simulink model "gimbal_test_2017_10_10"  (R2017a)
settings: Solver=ode14x  StartTime=0.0  StopTime=3  FixedStep=0.001  RelTol=1e-3  EnableMultiTasking=on
values from neighbouring files (symbols this model uses):
  m = MAG(:,3:5)    [acc_calibration_t1.m]
  s = tf('s')    [adaptive_control.m]    (also in constraints.m = 1e-19)
undefined symbols (not defined in the file or in its folder): sigbuilder_block, X, Y, Z
libraries: sm_lib x46, nesl_utility x29, simulink x7, sharedtransform x3
(part 2 of 2)

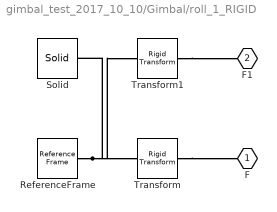
== system gimbal_test_2017_10_10/Gimbal/roll_1_RIGID ==
  ReferenceFrame : sm_lib/Frames and Transforms/Reference Frame
  Solid : sm_lib/Body Elements/Solid  InertiaType=Custom  Mass=0.31793228993235328  MassUnits=kg  CenterOfMass=[-40.197559372662035 151.39080125157062 -75.482343271011416]  CenterOfMassUnits=mm  MomentsOfInertia=[1698.578771208184 766.33943967936329 1161.8382457192142]  MomentsOfInertiaUnits=kg*mm^2  ProductsOfInertia=[-589.52899840909799 -20.442997774547614 -29.224073948839539]  ProductsOfInertiaUnits=kg*mm^2  DensityBased=on  Density=1000  DensityUnits=kg/(m^3)  DoExposeReferenceFrame=on  SerializedFrames=<Frames/>  GraphicType=FromGeometry  MarkerShape=Sphere  MarkerSize=10  GraphicVisPropType=SimpleVisualProperties  GraphicDiffuseColor=[0.89803921568627454 0.91764705882352937 0.92941176470588238]  GraphicSpecularColor=[0.5 0.5 0.5 1.0]  GraphicAmbientColor=[0.15 0.15 0.15 1.0]  GraphicEmissiveColor=[0.0 0.0 0.0 1.0]  GraphicShininess=75  GraphicOpacity=1  GeometryShape=FromFile  RectangleSize=[1 1]  RectangleSizeUnits=m  BrickDimensions=[1 1 1]  BrickDimensionUnits=m  CylinderRadius=1  CylinderRadiusUnits=m  CylinderLength=1  CylinderLengthUnits=m  SphereRadius=1  SphereRadiusUnits=m  EllipsoidRadii=[1 1 1]  EllipsoidRadiiUnits=m  ExtrusionCrossSection=[1 1; -1 1; -1 -1; 1 -1]  ExtrusionCrossSectionUnits=m  ExtrusionLength=1  ExtrusionLengthUnits=m  PolygonNumSides=3  PolygonOuterRadius=1  PolygonOuterRadiusUnits=m  ExtGeomFileType=STEP  ExtGeomFileName=roll_默认_sldprt.STEP  ExtGeomFileUnits=m  RevolutionCrossSection=[1 1; 1 -1; 2 -1; 2 1]  RevolutionCrossSectionUnits=m  RevolutionExtent=Full  RevolutionAngle=180  RevolutionAngleUnits=deg
  Transform : sm_lib/Frames and Transforms/Rigid Transform  TranslationMethod=Cartesian  TranslationStandardOffset=0  TranslationLengthUnit=mm  TranslationStandardAxis=+Z  TranslationCartesianOffset=[-38.909159672899136 47.175725301000313 513.35498149905948]  TranslationROffset=0  TranslationROffsetUnits=m  TranslationZOffset=0  TranslationZOffsetUnits=m  TranslationThetaOffset=0  TranslationThetaOffsetUnits=deg  RotationMethod=ArbitraryAxis  RotationAngleUnits=rad  RotationStandardAxis=+Z  RotationAngle=3.1415926535897931  RotationArbitraryAxis=[-1 1.5338031114433573e-32 -2.7175667253946204e-16]  FollAlignAxisA=+X  BaseAlignAxisA=+Y  FollAlignAxisB=+Y  BaseAlignAxisB=+Z  RotationSequenceAxes=FollowerAxes  RotationSequence=XYX  RotationSequenceAngles=[0 0 0]  RotationSequenceAnglesUnits=deg  RotationMatrix=[1 0 0; 0 1 0; 0 0 1]
  Transform1 : sm_lib/Frames and Transforms/Rigid Transform  TranslationMethod=Cartesian  TranslationStandardOffset=0  TranslationLengthUnit=mm  TranslationStandardAxis=+Z  TranslationCartesianOffset=[-38.909159672900039 1167.1810510685002 -32.030390597700006]  TranslationROffset=0  TranslationROffsetUnits=m  TranslationZOffset=0  TranslationZOffsetUnits=m  TranslationThetaOffset=0  TranslationThetaOffsetUnits=deg  RotationMethod=ArbitraryAxis  RotationAngleUnits=rad  RotationStandardAxis=+Z  RotationAngle=2.0943951023931953  RotationArbitraryAxis=[0.57735026918962584 -0.57735026918962584 0.57735026918962584]  FollAlignAxisA=+X  BaseAlignAxisA=+Y  FollAlignAxisB=+Y  BaseAlignAxisB=+Z  RotationSequenceAxes=FollowerAxes  RotationSequence=XYX  RotationSequenceAngles=[0 0 0]  RotationSequenceAnglesUnits=deg  RotationMatrix=[1 0 0; 0 1 0; 0 0 1]
  F : PMIOPort  Port=1  Side=Left
  F1 : PMIOPort  Port=2  Side=Right
  connections:
  Solid/RConn1 -- ReferenceFrame/RConn1 -- Transform/LConn1 -- Transform1/LConn1
  Transform/RConn1 -- F/RConn1
  Transform1/RConn1 -- F1/RConn1

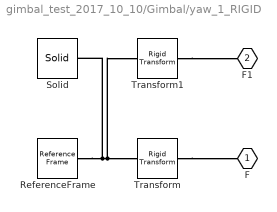
== system gimbal_test_2017_10_10/Gimbal/yaw_1_RIGID ==
  ReferenceFrame : sm_lib/Frames and Transforms/Reference Frame
  Solid : sm_lib/Body Elements/Solid  InertiaType=Custom  Mass=0.4220224652422469  MassUnits=kg  CenterOfMass=[-39.730395407906954 147.5203430562342 -125.35459490281445]  CenterOfMassUnits=mm  MomentsOfInertia=[6109.2729904538583 920.66918616811347 5510.6384164735264]  MomentsOfInertiaUnits=kg*mm^2  ProductsOfInertia=[-1282.9600428246124 21.67357327564007 52.078346871971853]  ProductsOfInertiaUnits=kg*mm^2  DensityBased=on  Density=1000  DensityUnits=kg/(m^3)  DoExposeReferenceFrame=on  SerializedFrames=<Frames/>  GraphicType=FromGeometry  MarkerShape=Sphere  MarkerSize=10  GraphicVisPropType=SimpleVisualProperties  GraphicDiffuseColor=[0.89803921568627454 0.91764705882352937 0.92941176470588238]  GraphicSpecularColor=[0.5 0.5 0.5 1.0]  GraphicAmbientColor=[0.15 0.15 0.15 1.0]  GraphicEmissiveColor=[0.0 0.0 0.0 1.0]  GraphicShininess=75  GraphicOpacity=1  GeometryShape=FromFile  RectangleSize=[1 1]  RectangleSizeUnits=m  BrickDimensions=[1 1 1]  BrickDimensionUnits=m  CylinderRadius=1  CylinderRadiusUnits=m  CylinderLength=1  CylinderLengthUnits=m  SphereRadius=1  SphereRadiusUnits=m  EllipsoidRadii=[1 1 1]  EllipsoidRadiiUnits=m  ExtrusionCrossSection=[1 1; -1 1; -1 -1; 1 -1]  ExtrusionCrossSectionUnits=m  ExtrusionLength=1  ExtrusionLengthUnits=m  PolygonNumSides=3  PolygonOuterRadius=1  PolygonOuterRadiusUnits=m  ExtGeomFileType=STEP  ExtGeomFileName=yaw_默认_sldprt.STEP  ExtGeomFileUnits=m  RevolutionCrossSection=[1 1; 1 -1; 2 -1; 2 1]  RevolutionCrossSectionUnits=m  RevolutionExtent=Full  RevolutionAngle=180  RevolutionAngleUnits=deg
  Transform : sm_lib/Frames and Transforms/Rigid Transform  TranslationMethod=Cartesian  TranslationStandardOffset=0  TranslationLengthUnit=mm  TranslationStandardAxis=+Z  TranslationCartesianOffset=[-38.909159672899804 334.03951901900109 -32.030390597700091]  TranslationROffset=0  TranslationROffsetUnits=m  TranslationZOffset=0  TranslationZOffsetUnits=m  TranslationThetaOffset=0  TranslationThetaOffsetUnits=deg  RotationMethod=ArbitraryAxis  RotationAngleUnits=rad  RotationStandardAxis=+Z  RotationAngle=2.0943951023931962  RotationArbitraryAxis=[0.57735026918962595 -0.57735026918962562 0.57735026918962573]  FollAlignAxisA=+X  BaseAlignAxisA=+Y  FollAlignAxisB=+Y  BaseAlignAxisB=+Z  RotationSequenceAxes=FollowerAxes  RotationSequence=XYX  RotationSequenceAngles=[0 0 0]  RotationSequenceAnglesUnits=deg  RotationMatrix=[1 0 0; 0 1 0; 0 0 1]
  Transform1 : sm_lib/Frames and Transforms/Rigid Transform  TranslationMethod=Cartesian  TranslationStandardOffset=0  TranslationLengthUnit=mm  TranslationStandardAxis=+Z  TranslationCartesianOffset=[-38.909159672900067 32.039519019000039 520.28895609530014]  TranslationROffset=0  TranslationROffsetUnits=m  TranslationZOffset=0  TranslationZOffsetUnits=m  TranslationThetaOffset=0  TranslationThetaOffsetUnits=deg  RotationMethod=ArbitraryAxis  RotationAngleUnits=rad  RotationStandardAxis=+Z  RotationAngle=3.1415926535897931  RotationArbitraryAxis=[1 0 5.377642775528102e-17]  FollAlignAxisA=+X  BaseAlignAxisA=+Y  FollAlignAxisB=+Y  BaseAlignAxisB=+Z  RotationSequenceAxes=FollowerAxes  RotationSequence=XYX  RotationSequenceAngles=[0 0 0]  RotationSequenceAnglesUnits=deg  RotationMatrix=[1 0 0; 0 1 0; 0 0 1]
  F : PMIOPort  Port=1  Side=Left
  F1 : PMIOPort  Port=2  Side=Right
  connections:
  Solid/RConn1 -- ReferenceFrame/RConn1 -- Transform/LConn1 -- Transform1/LConn1
  Transform/RConn1 -- F/RConn1
  Transform1/RConn1 -- F1/RConn1

== system gimbal_test_2017_10_10/Subsystem1/groud_1_RIGID ==
  ReferenceFrame : sm_lib/Frames and Transforms/Reference Frame
  Solid : sm_lib/Body Elements/Solid  InertiaType=Custom  Mass=0.744656095436107  MassUnits=kg  CenterOfMass=[0 14.834199182049298 0]  CenterOfMassUnits=mm  MomentsOfInertia=[248.52962199765179 383.88524366097863 245.75166872905808]  MomentsOfInertiaUnits=kg*mm^2  ProductsOfInertia=[0 0 0]  ProductsOfInertiaUnits=kg*mm^2  DensityBased=on  Density=1000  DensityUnits=kg/(m^3)  DoExposeReferenceFrame=on  SerializedFrames=<Frames/>  GraphicType=FromGeometry  MarkerShape=Sphere  MarkerSize=10  GraphicVisPropType=SimpleVisualProperties  GraphicDiffuseColor=[0.89411764705882346 0.9137254901960784 0.92941176470588238]  GraphicSpecularColor=[0.5 0.5 0.5 1.0]  GraphicAmbientColor=[0.15 0.15 0.15 1.0]  GraphicEmissiveColor=[0.0 0.0 0.0 1.0]  GraphicShininess=75  GraphicOpacity=1  GeometryShape=FromFile  RectangleSize=[1 1]  RectangleSizeUnits=m  BrickDimensions=[1 1 1]  BrickDimensionUnits=m  CylinderRadius=1  CylinderRadiusUnits=m  CylinderLength=1  CylinderLengthUnits=m  SphereRadius=1  SphereRadiusUnits=m  EllipsoidRadii=[1 1 1]  EllipsoidRadiiUnits=m  ExtrusionCrossSection=[1 1; -1 1; -1 -1; 1 -1]  ExtrusionCrossSectionUnits=m  ExtrusionLength=1  ExtrusionLengthUnits=m  PolygonNumSides=3  PolygonOuterRadius=1  PolygonOuterRadiusUnits=m  ExtGeomFileType=STEP  ExtGeomFileName=groud_默认_sldprt.STEP  ExtGeomFileUnits=m  RevolutionCrossSection=[1 1; 1 -1; 2 -1; 2 1]  RevolutionCrossSectionUnits=m  RevolutionExtent=Full  RevolutionAngle=180  RevolutionAngleUnits=deg
  Transform : sm_lib/Frames and Transforms/Rigid Transform  TranslationMethod=Cartesian  TranslationStandardOffset=0  TranslationLengthUnit=mm  TranslationStandardAxis=+Z  TranslationCartesianOffset=[0 30 0]  TranslationROffset=0  TranslationROffsetUnits=m  TranslationZOffset=0  TranslationZOffsetUnits=m  TranslationThetaOffset=0  TranslationThetaOffsetUnits=deg  RotationMethod=ArbitraryAxis  RotationAngleUnits=rad  RotationStandardAxis=+Z  RotationAngle=2.0943951023931953  RotationArbitraryAxis=[0.57735026918962584 -0.57735026918962584 0.57735026918962584]  FollAlignAxisA=+X  BaseAlignAxisA=+Y  FollAlignAxisB=+Y  BaseAlignAxisB=+Z  RotationSequenceAxes=FollowerAxes  RotationSequence=XYX  RotationSequenceAngles=[0 0 0]  RotationSequenceAnglesUnits=deg  RotationMatrix=[1 0 0; 0 1 0; 0 0 1]
  F1 : PMIOPort  Port=1  Side=Left
  F : PMIOPort  Port=2  Side=Right
  connections:
  Solid/RConn1 -- ReferenceFrame/RConn1 -- Transform/LConn1 -- F1/RConn1
  Transform/RConn1 -- F/RConn1

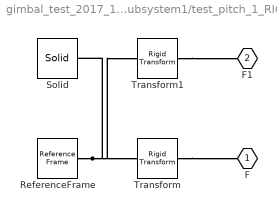
== system gimbal_test_2017_10_10/Subsystem1/test_pitch_1_RIGID ==
  ReferenceFrame : sm_lib/Frames and Transforms/Reference Frame
  Solid : sm_lib/Body Elements/Solid  InertiaType=Custom  Mass=3.2542558482698221  MassUnits=kg  CenterOfMass=[0 15.000000000000004 0.00013445046945364221]  CenterOfMassUnits=mm  MomentsOfInertia=[197323.97689125084 354318.98035563418 157585.85549691919]  MomentsOfInertiaUnits=kg*mm^2  ProductsOfInertia=[0 0 0.0039657370023979469]  ProductsOfInertiaUnits=kg*mm^2  DensityBased=on  Density=1000  DensityUnits=kg/(m^3)  DoExposeReferenceFrame=on  SerializedFrames=<Frames/>  GraphicType=FromGeometry  MarkerShape=Sphere  MarkerSize=10  GraphicVisPropType=SimpleVisualProperties  GraphicDiffuseColor=[1 1 1]  GraphicSpecularColor=[0.5 0.5 0.5 1.0]  GraphicAmbientColor=[0.15 0.15 0.15 1.0]  GraphicEmissiveColor=[0.0 0.0 0.0 1.0]  GraphicShininess=75  GraphicOpacity=1  GeometryShape=FromFile  RectangleSize=[1 1]  RectangleSizeUnits=m  BrickDimensions=[1 1 1]  BrickDimensionUnits=m  CylinderRadius=1  CylinderRadiusUnits=m  CylinderLength=1  CylinderLengthUnits=m  SphereRadius=1  SphereRadiusUnits=m  EllipsoidRadii=[1 1 1]  EllipsoidRadiiUnits=m  ExtrusionCrossSection=[1 1; -1 1; -1 -1; 1 -1]  ExtrusionCrossSectionUnits=m  ExtrusionLength=1  ExtrusionLengthUnits=m  PolygonNumSides=3  PolygonOuterRadius=1  PolygonOuterRadiusUnits=m  ExtGeomFileType=STEP  ExtGeomFileName=test_pitch_默认_sldprt.STEP  ExtGeomFileUnits=m  RevolutionCrossSection=[1 1; 1 -1; 2 -1; 2 1]  RevolutionCrossSectionUnits=m  RevolutionExtent=Full  RevolutionAngle=180  RevolutionAngleUnits=deg
  Transform : sm_lib/Frames and Transforms/Rigid Transform  TranslationMethod=Cartesian  TranslationStandardOffset=0  TranslationLengthUnit=mm  TranslationStandardAxis=+Z  TranslationCartesianOffset=[0 15.000000000000568 -587]  TranslationROffset=0  TranslationROffsetUnits=m  TranslationZOffset=0  TranslationZOffsetUnits=m  TranslationThetaOffset=0  TranslationThetaOffsetUnits=deg  RotationMethod=ArbitraryAxis  RotationAngleUnits=rad  RotationStandardAxis=+Z  RotationAngle=8.3312973296909746e-16  RotationArbitraryAxis=[0.86265645032380789 -0.50579032089861853 -1.8175695005807099e-16]  FollAlignAxisA=+X  BaseAlignAxisA=+Y  FollAlignAxisB=+Y  BaseAlignAxisB=+Z  RotationSequenceAxes=FollowerAxes  RotationSequence=XYX  RotationSequenceAngles=[0 0 0]  RotationSequenceAnglesUnits=deg  RotationMatrix=[1 0 0; 0 1 0; 0 0 1]
  Transform1 : sm_lib/Frames and Transforms/Rigid Transform  TranslationMethod=Cartesian  TranslationStandardOffset=0  TranslationLengthUnit=mm  TranslationStandardAxis=+Z  TranslationCartesianOffset=[0 30 0]  TranslationROffset=0  TranslationROffsetUnits=m  TranslationZOffset=0  TranslationZOffsetUnits=m  TranslationThetaOffset=0  TranslationThetaOffsetUnits=deg  RotationMethod=ArbitraryAxis  RotationAngleUnits=rad  RotationStandardAxis=+Z  RotationAngle=2.0943951023931953  RotationArbitraryAxis=[0.57735026918962584 -0.57735026918962584 0.57735026918962584]  FollAlignAxisA=+X  BaseAlignAxisA=+Y  FollAlignAxisB=+Y  BaseAlignAxisB=+Z  RotationSequenceAxes=FollowerAxes  RotationSequence=XYX  RotationSequenceAngles=[0 0 0]  RotationSequenceAnglesUnits=deg  RotationMatrix=[1 0 0; 0 1 0; 0 0 1]
  F : PMIOPort  Port=1  Side=Left
  F1 : PMIOPort  Port=2  Side=Right
  connections:
  Solid/RConn1 -- ReferenceFrame/RConn1 -- Transform/LConn1 -- Transform1/LConn1
  Transform/RConn1 -- F/RConn1
  Transform1/RConn1 -- F1/RConn1

== system gimbal_test_2017_10_10/Subsystem1/test_roll_1_RIGID ==
  ReferenceFrame : sm_lib/Frames and Transforms/Reference Frame
  Solid : sm_lib/Body Elements/Solid  InertiaType=Custom  Mass=0.20450614916336574  MassUnits=kg  CenterOfMass=[-1.0328761560106987e-05 10.226639389930648 -309.12731029151979]  CenterOfMassUnits=mm  MomentsOfInertia=[71.504553359544801 477.13713336271184 448.94842380562415]  MomentsOfInertiaUnits=kg*mm^2  ProductsOfInertia=[-0.44644966825853433 2.6790546083628789e-05 -3.8747955667632615e-05]  ProductsOfInertiaUnits=kg*mm^2  DensityBased=on  Density=1000  DensityUnits=kg/(m^3)  DoExposeReferenceFrame=on  SerializedFrames=<Frames/>  GraphicType=FromGeometry  MarkerShape=Sphere  MarkerSize=10  GraphicVisPropType=SimpleVisualProperties  GraphicDiffuseColor=[1 1 1]  GraphicSpecularColor=[0.5 0.5 0.5 1.0]  GraphicAmbientColor=[0.15 0.15 0.15 1.0]  GraphicEmissiveColor=[0.0 0.0 0.0 1.0]  GraphicShininess=75  GraphicOpacity=1  GeometryShape=FromFile  RectangleSize=[1 1]  RectangleSizeUnits=m  BrickDimensions=[1 1 1]  BrickDimensionUnits=m  CylinderRadius=1  CylinderRadiusUnits=m  CylinderLength=1  CylinderLengthUnits=m  SphereRadius=1  SphereRadiusUnits=m  EllipsoidRadii=[1 1 1]  EllipsoidRadiiUnits=m  ExtrusionCrossSection=[1 1; -1 1; -1 -1; 1 -1]  ExtrusionCrossSectionUnits=m  ExtrusionLength=1  ExtrusionLengthUnits=m  PolygonNumSides=3  PolygonOuterRadius=1  PolygonOuterRadiusUnits=m  ExtGeomFileType=STEP  ExtGeomFileName=test_roll_默认_sldprt.STEP  ExtGeomFileUnits=m  RevolutionCrossSection=[1 1; 1 -1; 2 -1; 2 1]  RevolutionCrossSectionUnits=m  RevolutionExtent=Full  RevolutionAngle=180  RevolutionAngleUnits=deg
  Transform : sm_lib/Frames and Transforms/Rigid Transform  TranslationMethod=Cartesian  TranslationStandardOffset=0  TranslationLengthUnit=mm  TranslationStandardAxis=+Z  TranslationCartesianOffset=[8.9090429904744592e-15 1.0221477966047367e-13 -1.1911909021789691e-13]  TranslationROffset=0  TranslationROffsetUnits=m  TranslationZOffset=0  TranslationZOffsetUnits=m  TranslationThetaOffset=0  TranslationThetaOffsetUnits=deg  RotationMethod=ArbitraryAxis  RotationAngleUnits=rad  RotationStandardAxis=+Z  RotationAngle=2.0943951023931953  RotationArbitraryAxis=[0.57735026918962584 -0.57735026918962629 0.57735026918962529]  FollAlignAxisA=+X  BaseAlignAxisA=+Y  FollAlignAxisB=+Y  BaseAlignAxisB=+Z  RotationSequenceAxes=FollowerAxes  RotationSequence=XYX  RotationSequenceAngles=[0 0 0]  RotationSequenceAnglesUnits=deg  RotationMatrix=[1 0 0; 0 1 0; 0 0 1]
  Transform1 : sm_lib/Frames and Transforms/Rigid Transform  TranslationMethod=Cartesian  TranslationStandardOffset=0  TranslationLengthUnit=mm  TranslationStandardAxis=+Z  TranslationCartesianOffset=[14.999999999999972 9.9999999999999947 -299.99999999999983]  TranslationROffset=0  TranslationROffsetUnits=m  TranslationZOffset=0  TranslationZOffsetUnits=m  TranslationThetaOffset=0  TranslationThetaOffsetUnits=deg  RotationMethod=ArbitraryAxis  RotationAngleUnits=rad  RotationStandardAxis=+Z  RotationAngle=0  RotationArbitraryAxis=[0 0 0]  FollAlignAxisA=+X  BaseAlignAxisA=+Y  FollAlignAxisB=+Y  BaseAlignAxisB=+Z  RotationSequenceAxes=FollowerAxes  RotationSequence=XYX  RotationSequenceAngles=[0 0 0]  RotationSequenceAnglesUnits=deg  RotationMatrix=[1 0 0; 0 1 0; 0 0 1]
  F1 : PMIOPort  Port=1  Side=Left
  F : PMIOPort  Port=2  Side=Left
  connections:
  Solid/RConn1 -- ReferenceFrame/RConn1 -- Transform/LConn1 -- Transform1/LConn1
  Transform/RConn1 -- F/RConn1
  Transform1/RConn1 -- F1/RConn1

== system gimbal_test_2017_10_10/Subsystem1/test_yaw_1_RIGID ==
  ReferenceFrame : sm_lib/Frames and Transforms/Reference Frame
  Solid : sm_lib/Body Elements/Solid  InertiaType=Custom  Mass=1.613673260827966  MassUnits=kg  CenterOfMass=[-248.89867877972853 25.000221887150591 -0.00036630926726364301]  CenterOfMassUnits=mm  MomentsOfInertia=[104081.22099303995 121622.83981515096 18191.454171364006]  MomentsOfInertiaUnits=kg*mm^2  ProductsOfInertia=[-0.001740744498014553 0.078222601983178194 -0.083617721522158003]  ProductsOfInertiaUnits=kg*mm^2  DensityBased=on  Density=1000  DensityUnits=kg/(m^3)  DoExposeReferenceFrame=on  SerializedFrames=<Frames/>  GraphicType=FromGeometry  MarkerShape=Sphere  MarkerSize=10  GraphicVisPropType=SimpleVisualProperties  GraphicDiffuseColor=[1 1 1]  GraphicSpecularColor=[0.5 0.5 0.5 1.0]  GraphicAmbientColor=[0.15 0.15 0.15 1.0]  GraphicEmissiveColor=[0.0 0.0 0.0 1.0]  GraphicShininess=75  GraphicOpacity=1  GeometryShape=FromFile  RectangleSize=[1 1]  RectangleSizeUnits=m  BrickDimensions=[1 1 1]  BrickDimensionUnits=m  CylinderRadius=1  CylinderRadiusUnits=m  CylinderLength=1  CylinderLengthUnits=m  SphereRadius=1  SphereRadiusUnits=m  EllipsoidRadii=[1 1 1]  EllipsoidRadiiUnits=m  ExtrusionCrossSection=[1 1; -1 1; -1 -1; 1 -1]  ExtrusionCrossSectionUnits=m  ExtrusionLength=1  ExtrusionLengthUnits=m  PolygonNumSides=3  PolygonOuterRadius=1  PolygonOuterRadiusUnits=m  ExtGeomFileType=STEP  ExtGeomFileName=test_yaw_默认_sldprt.STEP  ExtGeomFileUnits=m  RevolutionCrossSection=[1 1; 1 -1; 2 -1; 2 1]  RevolutionCrossSectionUnits=m  RevolutionExtent=Full  RevolutionAngle=180  RevolutionAngleUnits=deg
  Transform : sm_lib/Frames and Transforms/Rigid Transform  TranslationMethod=Cartesian  TranslationStandardOffset=0  TranslationLengthUnit=mm  TranslationStandardAxis=+Z  TranslationCartesianOffset=[0 24.999999999999968 -587]  TranslationROffset=0  TranslationROffsetUnits=m  TranslationZOffset=0  TranslationZOffsetUnits=m  TranslationThetaOffset=0  TranslationThetaOffsetUnits=deg  RotationMethod=ArbitraryAxis  RotationAngleUnits=rad  RotationStandardAxis=+Z  RotationAngle=0  RotationArbitraryAxis=[0 0 0]  FollAlignAxisA=+X  BaseAlignAxisA=+Y  FollAlignAxisB=+Y  BaseAlignAxisB=+Z  RotationSequenceAxes=FollowerAxes  RotationSequence=XYX  RotationSequenceAngles=[0 0 0]  RotationSequenceAnglesUnits=deg  RotationMatrix=[1 0 0; 0 1 0; 0 0 1]
  Transform1 : sm_lib/Frames and Transforms/Rigid Transform  TranslationMethod=Cartesian  TranslationStandardOffset=0  TranslationLengthUnit=mm  TranslationStandardAxis=+Z  TranslationCartesianOffset=[-425.19949180560275 25.000000000000032 -5.6843418860808015e-14]  TranslationROffset=0  TranslationROffsetUnits=m  TranslationZOffset=0  TranslationZOffsetUnits=m  TranslationThetaOffset=0  TranslationThetaOffsetUnits=deg  RotationMethod=ArbitraryAxis  RotationAngleUnits=rad  RotationStandardAxis=+Z  RotationAngle=2.0943951023931953  RotationArbitraryAxis=[0.57735026918962562 0.57735026918962562 0.57735026918962595]  FollAlignAxisA=+X  BaseAlignAxisA=+Y  FollAlignAxisB=+Y  BaseAlignAxisB=+Z  RotationSequenceAxes=FollowerAxes  RotationSequence=XYX  RotationSequenceAngles=[0 0 0]  RotationSequenceAnglesUnits=deg  RotationMatrix=[1 0 0; 0 1 0; 0 0 1]
  F1 : PMIOPort  Port=1  Side=Left
  F : PMIOPort  Port=2  Side=Right
  connections:
  Solid/RConn1 -- ReferenceFrame/RConn1 -- Transform/LConn1 -- Transform1/LConn1
  Transform/RConn1 -- F/RConn1
  Transform1/RConn1 -- F1/RConn1

== matlab function gimbal_test_2017_10_10/MATLAB Function1 ==
  data: A input; y output; Rot input
function y = fcn(A, Rot)

y = Rot*A;

== matlab function gimbal_test_2017_10_10/MATLAB Function ==
  data: vel_fb output; enc input; gyro input
function vel_fb = speed_fb(enc, gyro)
vr_fb = cos(enc(2))*gyro(1) + sin(enc(2))*gyro(3);
vp_fb = sin(enc(2))*tan(enc(1))*gyro(1) + gyro(2) + cos(enc(2))*tan(enc(1))*gyro(3);
vy_fb = sin(-enc(2))*gyro(1)/cos(enc(1)) + cos(enc(2))*gyro(3)/cos(enc(1));
vel_fb = [vr_fb;vp_fb;vy_fb];

== matlab function gimbal_test_2017_10_10/pitch rot ==
  data: angle input; RM output
function RM = rot_pitch(angle)
%#codegen
RM = [cos(angle) 0 sin(angle);
      0          1 0;
      -sin(angle) 0 cos(angle);];

== matlab function gimbal_test_2017_10_10/Gimbal/Pitch Enc ==
  data: angle input; y output; bias input
function y = enc(angle, bias)
%#codegen
while angle>pi
    angle = angle - 2*pi;
end
while angle<-pi
    angle = angle + 2*pi;
end
angle = angle + bias;
if angle>pi
    angle = angle - 2*pi;
end
if angle<-pi
    angle = angle + 2*pi;
end
y = angle;

== matlab function gimbal_test_2017_10_10/Gimbal/Pitch Enc1 ==
  data: angle input; y output; bias input
function y = enc(angle, bias)
%#codegen
while angle>pi
    angle = angle - 2*pi;
end
while angle<-pi
    angle = angle + 2*pi;
end
angle = angle + bias;
if angle>pi
    angle = angle - 2*pi;
end
if angle<-pi
    angle = angle + 2*pi;
end
y = angle;

== matlab function gimbal_test_2017_10_10/Gimbal/Pitch Enc2 ==
  data: angle input; y output; bias input
function y = enc(angle, bias)
%#codegen
while angle>pi
    angle = angle - 2*pi;
end
while angle<-pi
    angle = angle + 2*pi;
end
angle = angle + bias;
if angle>pi
    angle = angle - 2*pi;
end
if angle<-pi
    angle = angle + 2*pi;
end
y = angle;

== matlab function gimbal_test_2017_10_10/roll rot1 ==
  data: angle input; RM output
function RM = rot_roll(angle)
%#codegen
RM = [1 0 0;
      0 cos(angle) -sin(angle);
      0 sin(angle) cos(angle);];

== matlab function gimbal_test_2017_10_10/MATLAB Function3 ==
  data: A input; y output; Rot input
function y = fcn(A, Rot)

y = Rot*A;

== matlab function gimbal_test_2017_10_10/roll rot ==
  data: angle input; RM output
function RM = rot_roll(angle)
%#codegen
RM = [1 0 0;
      0 cos(angle) -sin(angle);
      0 sin(angle) cos(angle);];

== matlab function gimbal_test_2017_10_10/yaw rot ==
  data: angle input; RM output
function RM = rot_roll(angle)
%#codegen
RM = [cos(angle) -sin(angle) 0;
      sin(angle) cos(angle) 0;
      0 0 1;];

== matlab function gimbal_test_2017_10_10/Camera IMU/MATLAB Function2 ==
  data: w input; gyro output; RM input
function gyro = fcn(w, RM)
%#codegen
gyro = inv(RM)*w;

== matlab function gimbal_test_2017_10_10/MATLAB Function2 ==
  data: A_dst input; mot_angle_out output; A_now input; enc input
function mot_angle_out = fcn(A_dst, A_now, enc)
sx = sin(enc(1));
cx = cos(enc(1));
sy = sin(enc(2));
cy = cos(enc(2));
sz = sin(enc(3));
cz = cos(enc(3));
T = [cz*cy-sz*sx*sy     -sz*cx     cz*sy+sz*sx*cy;
     sz*cy+cz*sx*sy     cz*cx      sz*sy-cz*sx*cy;
     -cx*sy             sx         cx*cy;];
T1 = T*pinv(A_now)*A_dst;
nx = T1(1,1);
ny = T1(2,1);
nz = T1(3,1);
ox = T1(1,2);
oy = T1(2,2);
oz = T1(3,2);
ax = T1(1,3);
ay = T1(2,3);
az = T1(3,3);

%电机目标角度
agz = atan2(-ox, oy);
agx = atan2(oz, oy*cos(agz)-ox*sin(agz));
agy = atan2(ax*cos(agz)+ay*sin(agz), nx*cos(agz)+ny*sin(agz));

mot_angle_out = [agx-enc(1); agy-enc(2); agz-enc(3)];

== matlab function gimbal_test_2017_10_10/MATLAB Function4 ==
  data: DCM_imu input; DCM_body output; enc input; track_z output
function [DCM_body,track_z] = fcn(DCM_imu,enc)
x = 0;
y = 0;
z = 0;
if length(enc)== 3
    x = -enc(1);
    y = -enc(2);
    z = -enc(3);
end
T = [cos(y)*cos(z)+sin(y)*sin(x)*sin(z)     -cos(y)*sin(z)+sin(y)*sin(x)*cos(z)      sin(y)*cos(x);
     cos(x)*sin(z)                          cos(x)*cos(z)                            -sin(x);
     -sin(y)*cos(z)+cos(y)*sin(x)*sin(z)    sin(y)*sin(z)+cos(y)*sin(x)*cos(z)       cos(y)*cos(x);];
 
 DCM_body = DCM_imu*T;
 
 track_z = atan2(DCM_body(2,1),DCM_body(1,1));

== matlab function gimbal_test_2017_10_10/Body IMU/MATLAB Function2 ==
  data: w input; gyro output; RM input
function gyro = fcn(w, RM)
%#codegen
gyro = inv(RM)*w;

== matlab function gimbal_test_2017_10_10/MATLAB Function5 ==
  data: q input; DCM output; ROT output; len_q output
function [DCM, ROT, len_q] = quat_dcm(q)
q0 = q(1);
q1 = q(2);
q2 = q(3);
q3 = q(4);
q00 = q0*q0;
q11 = q1*q1;
q22 = q2*q2;
q33 = q3*q3;
len_q = sqrt(q00+q11+q22+q33);
DCM = [q00 + q11 - q22 - q33  2*(q1*q2+q0*q3)  2*(q1*q3-q0*q2);
       2*(q1*q2-q0*q3)  q00 - q11 + q22 - q33  2*(q2*q3+q0*q1);
       2*(q1*q3+q0*q2)  2*(q2*q3-q0*q1)  q00 - q11 - q22 + q33;];

qr = q(1);
qi = q(2);
qj = q(3);
qk = q(4);
qii = qi*qi;
qjj = qj*qj;
qkk = qk*qk;
s = 1;%||q||^-2
ROT = [1-2*s*(qjj+qkk)      2*s*(qi*qj-qk*qr)       2*s*(qi*qk+qj*qr);
       2*s*(qi*qj+qk*qr)    1-2*s*(qii+qkk)         2*s*(qj*qk-qi*qr);
       2*s*(qi*qk-qj*qr)    2*s*(qj*qk+qi*qr)       1-2*s*(qii+qjj);];

== matlab function gimbal_test_2017_10_10/Subsystem/Quat body2earth ==
  data: quatb output; enc input
function quatb = quat_b2c(enc)
x2 = -enc(1)/2;
y2 = -enc(2)/2;
z2 = -enc(3)/2;
quat = zeros(1,4);
quat(1) = cos(z2)*cos(x2)*cos(y2) + sin(z2)*sin(x2)*sin(y2);
quat(2) = -cos(z2)*sin(x2)*cos(y2) - sin(z2)*cos(x2)*sin(y2);
quat(3) = -cos(z2)*cos(x2)*sin(y2) + sin(z2)*sin(x2)*cos(y2);
quat(4) = cos(z2)*sin(x2)*sin(y2) - sin(z2)*cos(x2)*cos(y2);
quatb = [quat(1) quat(2) quat(3) quat(4)];%quatmultiply(quat, quatc);

== matlab function gimbal_test_2017_10_10/Subsystem/quat product  ==
  data: a input; c output; b input
function c  = quat_pro(a, b)
c = zeros(1,4);
c(1) = a(1)*b(1) - a(2)*b(2) - a(3)*b(3) - a(4)*b(4);
c(2) = a(1)*b(2) + a(2)*b(1) + a(3)*b(4) - a(4)*b(3);
c(3) = a(1)*b(3) - a(2)*b(4) + a(3)*b(1) + a(4)*b(2);
c(4) = a(1)*b(4) + a(2)*b(3) - a(3)*b(2) + a(4)*b(1);

== matlab function gimbal_test_2017_10_10/conj  ==
  data: q input; cq output
function cq = fcn(q)
cq = zeros(1,4);
cq(1) = q(1);
cq(2) = -q(2);
cq(3) = -q(3);
cq(4) = -q(4);

== matlab function gimbal_test_2017_10_10/Subsystem/conj 1 ==
  data: q input; cq output
function cq = fcn(q)
cq = zeros(1,4);
cq(1) = q(1);
cq(2) = -q(2);
cq(3) = -q(3);
cq(4) = -q(4);

== matlab function gimbal_test_2017_10_10/Subsystem/conj 2 ==
  data: q input; cq output
function cq = fcn(q)
cq = zeros(1,4);
cq(1) = q(1);
cq(2) = -q(2);
cq(3) = -q(3);
cq(4) = -q(4);
